simulink model "EjemploSimulink"  (R2024b)
settings: Solver=VariableStepAuto  StartTime=0.0  StopTime=10.0  RelTol=1e-3
settings Model: Creator=user  LastModifiedBy=user

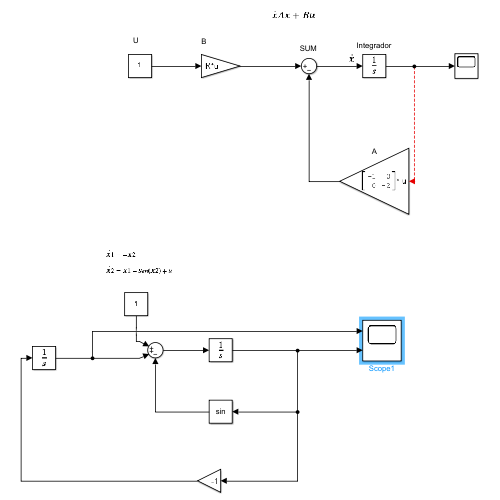
[thumbnail: Simulink's stored preview of the top-level diagram]
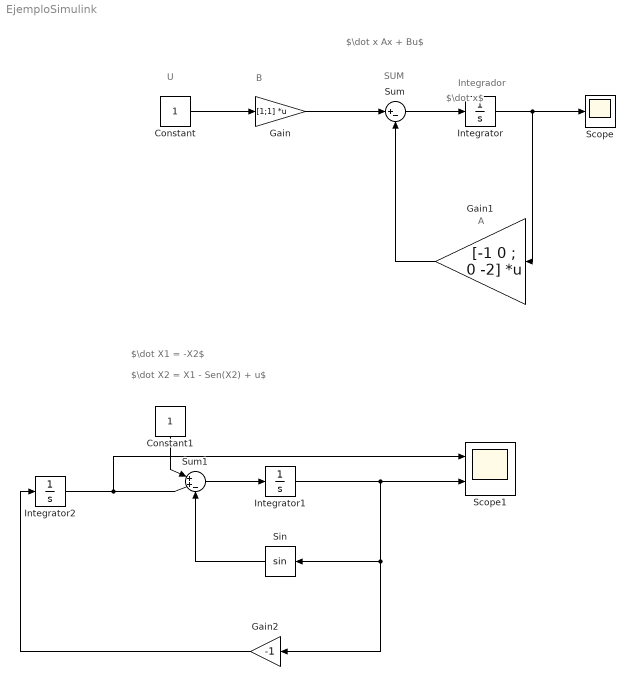
== system EjemploSimulink ==
  note: $\dot X2 = X1 - Sen(X2) + u$
  note: $\dot X1 = -X2$
  note: A
  note: Integrador
  note: $\dot x$
  note: SUM
  note: B
  note: U
  note: $\dot x Ax + Bu$
  Constant : Constant
  Constant1 : Constant
  Gain : Gain  Gain=[1;1]  Multiplication=Matrix(K*u)
  Gain1 : Gain  Gain=[-1 0 ; 0 -2]  Multiplication=Matrix(K*u)
  Gain2 : Gain  Gain=-1
  Integrator : Integrator  InitialCondition=[-1 ; 1]
  Integrator1 : Integrator
  Integrator2 : Integrator
  Scope : Scope
  Scope1 : Scope  NumInputPorts=2
  Sin : Trigonometry
  Sum : Sum  Inputs=|+-
  Sum1 : Sum  Inputs=|++-
  wires:
  Constant/1 -> Gain/1
  Gain/1 -> Sum/1
  Sum/1 -> Integrator/1
  Integrator/1 -> Gain1/1, Scope/1
  Gain1/1 -> Sum/2
  Constant1/1 -> Sum1/1
  Sum1/1 -> Integrator1/1
  Integrator1/1 -> Gain2/1, Sin/1, Scope1/2
  Sin/1 -> Sum1/3
  Gain2/1 -> Integrator2/1
  Integrator2/1 -> Scope1/1, Sum1/2
